simulink model "IdealVS_RL2"  (R2017a)
settings: Solver=ode45  StartTime=0.0  StopTime=0.1  RelTol=1e-3
libraries: fl_lib x7, nesl_utility x4
settings Model: Creator=mmi-vsa  LastModifiedBy=acs-mmi
settings DataIOCC: LimitDataPoints=on  SaveFormat=Array
settings OptimizationCC: BlockReduction=off  BooleanDataType=off  LifeSpan=inf
settings DebuggingCC: SaveWithParameterizedLinksMsg=none  UnderspecifiedInitializationDetection=Classic  MergeDetectMultiDrivingBlocksExec=none  SignalResolutionControl=TryResolveAllWithWarning  SFUnexpectedBacktrackingDiag=warning  SFNoUnconditionalDefaultTransitionDiag=warning  SFExecutionAtInitializationDiag=none
settings HardwareCC: ProdBitPerPointer=32  ProdBitPerSizeT=32  ProdBitPerPtrDiffT=32  ProdLargestAtomicFloat=None  ProdIntDivRoundTo=Undefined  ProdEndianess=Unspecified  ProdWordSize=32  ProdHWDeviceType=32-bit Generic  TargetUnknown=on
settings ModelReferenceCC: PropagateSignalLabelsOutOfModel=off
settings GRTTargetCC: TargetLangStandard=C89/C90 (ANSI)  GeneratePreprocessorConditionals=Disable all
settings ConfigComp: CovMetricSettings=dw  CovHtmlReporting=on  CovSaveCumulativeToWorkspaceVar=on  CovSaveSingleToWorkspaceVar=on  CovExternalEMLEnable=off  CovSFcnEnable=off

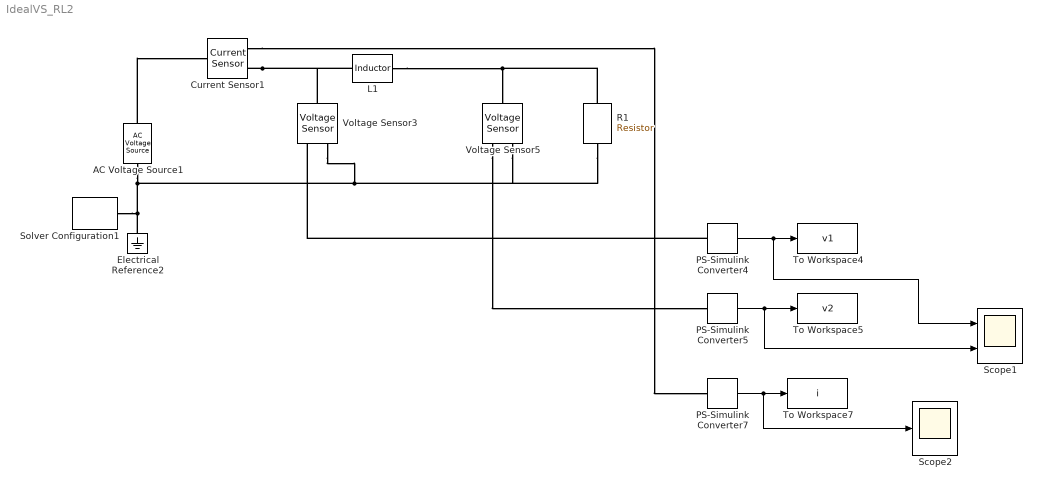
== system IdealVS_RL2 ==
  AC Voltage Source1 : fl_lib/Electrical/Electrical Sources/AC Voltage Source  amp=100 V  shift=90 deg  frequency=50 Hz  omega=0 rad/s
  Current Sensor1 : fl_lib/Electrical/Electrical Sensors/Current Sensor
  Electrical Reference2 : fl_lib/Electrical/Electrical Elements/Electrical Reference
  L1 : fl_lib/Electrical/Electrical Elements/Inductor  l=0.001 H  r=0 Ohm  g=0 1/Ohm  i_specify=off  i_priority=High  i=0 A  i_nominal_specify=off  i_nominal_unit=A  i_nominal_value=1  v_specify=off  v_priority=High  v=0 V  v_nominal_specify=off  v_nominal_unit=V  v_nominal_value=1  i_L_specify=off  i_L_priority=High  i_L=0 A  i_L_nominal_specify=off  i_L_nominal_unit=A  i_L_nominal_value=1
  PS-Simulink Converter4 : nesl_utility/PS-Simulink Converter  PhysicalDomain=network_engine_domain  SubClassName=ps_output  LeftPortType=input  RightPortType=output  PseudoPeriodic=off  Frequencies=[]  Unit=1  AffineConversion=off
  PS-Simulink Converter5 : nesl_utility/PS-Simulink Converter  PhysicalDomain=network_engine_domain  SubClassName=ps_output  LeftPortType=input  RightPortType=output  PseudoPeriodic=off  Frequencies=[]  Unit=1  AffineConversion=off
  PS-Simulink Converter7 : nesl_utility/PS-Simulink Converter  PhysicalDomain=network_engine_domain  SubClassName=ps_output  LeftPortType=input  RightPortType=output  PseudoPeriodic=off  Frequencies=[]  Unit=1  AffineConversion=off
  R1 : fl_lib/Electrical/Electrical Elements/Resistor  R=1 Ohm  i_specify=off  i_priority=High  i=0 A  i_nominal_specify=off  i_nominal_unit=A  i_nominal_value=1  v_specify=off  v_priority=High  v=0 V  v_nominal_specify=off  v_nominal_unit=V  v_nominal_value=1
  Scope1 : Scope  NumInputPorts=2
  Scope2 : Scope
  Solver Configuration1 : nesl_utility/Solver Configuration  PhysicalDomain=network_engine_domain  SubClassName=solver  LeftPortType=input  RightPortType=generic  Accelerate=off  Tones=[]  Harmonics=[]  SimulateNoise=off  Profile=off  UseLocalSampling=off  EnableSwitchedLinearOptims=on  FrequencyDomain=off  UseCCode=off  RelTol=0.001  AbsTol=1e-06  MinStep=1e-09  ToWorkspace=off  RevertToSquareIcSolve=off  NumHomotopyIterations=100  PhasorMode=off  PhasorModeNumHarmonics=1  OverrideAbsTol=off  DoDC=off  ResidualTolerance=1e-09  UseLocalSolver=on  LocalSolverChoice=NE_TRAPEZOIDAL_ADVANCER  LocalSolverSampleTime=5e-5  DoFixedCost=on  MaxNonlinIter=3  MaxModeIter=2  LinearAlgebra=Sparse  DelaysMemoryBudget=1024  AutomaticFiltering=on  FilteringTimeConstant=0.001
  To Workspace4 : ToWorkspace  VariableName=v1  SampleTime=-1
  To Workspace5 : ToWorkspace  VariableName=v2  SampleTime=-1
  To Workspace7 : ToWorkspace  VariableName=i  SampleTime=-1
  Voltage Sensor3 : fl_lib/Electrical/Electrical Sensors/Voltage Sensor
  Voltage Sensor5 : fl_lib/Electrical/Electrical Sensors/Voltage Sensor
  wires:
  PS-Simulink Converter4/1 -> Scope1/1, To Workspace4/1
  PS-Simulink Converter7/1 -> Scope2/1, To Workspace7/1
  PS-Simulink Converter5/1 -> Scope1/2, To Workspace5/1
  connections:
  Current Sensor1/RConn2 -- Voltage Sensor3/LConn1 -- L1/LConn1
  R1/LConn1 -- L1/RConn1 -- Voltage Sensor5/LConn1
  AC Voltage Source1/LConn1 -- Current Sensor1/LConn1
  PS-Simulink Converter4/LConn1 -- Voltage Sensor3/RConn1
  Voltage Sensor5/RConn1 -- PS-Simulink Converter5/LConn1
  Current Sensor1/RConn1 -- PS-Simulink Converter7/LConn1
  Electrical Reference2/LConn1 -- Voltage Sensor5/RConn2 -- R1/RConn1 -- Voltage Sensor3/RConn2 -- AC Voltage Source1/RConn1 -- Solver Configuration1/RConn1
